simulink model "Guardian_Battery_ECM"  (R2025b)
settings: Solver=FixedStepDiscrete  StartTime=0.0  StopTime=3600  FixedStep=1  MaxStep=1  RelTol=1e-3
values from neighbouring files (symbols this model uses):
  C1 = 17000    [EKF_SOC_Estimator.m]    (also in Guardian_inputs.m)
  C2 = 5200    [Guardian_inputs.m]
  FilterDenominator = [1 -0.98]    [Guardian_inputs.m]
  FilterNumerator = [0.02]    [Guardian_inputs.m]
  NoiseLower = -0.005    [Guardian_inputs.m]
  NoiseUpper = 0.005    [Guardian_inputs.m]
  OCV_V = OCV_Table.OCV_V    [Guardian_inputs.m]
  Q_nominal = 50    [Guardian_inputs.m]
  R0 = 0.00070    (= 0.0007)    [EKF_SOC_Estimator.m]    (also in Guardian_inputs.m)
  R1 = 0.00160    (= 0.0016)    [EKF_SOC_Estimator.m]    (also in Guardian_inputs.m)
  R2 = 0.00035    [Guardian_inputs.m]
  SOC_initial = 80    [Guardian_inputs.m]
  SOC_pct = OCV_Table.SOC_pct    [Guardian_inputs.m]
  Ts = 1    [Guardian_inputs.m]
undefined symbols (not defined in the file or in its folder): dspblkCoreblockFVToolHelper, gcbh
libraries: simulink x1
settings Model: Creator=ENJAZ  LastModifiedBy=ENJAZ

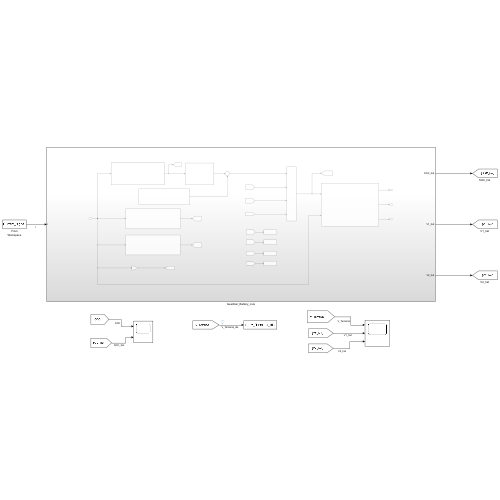
[thumbnail: Simulink's stored preview of the top-level diagram]
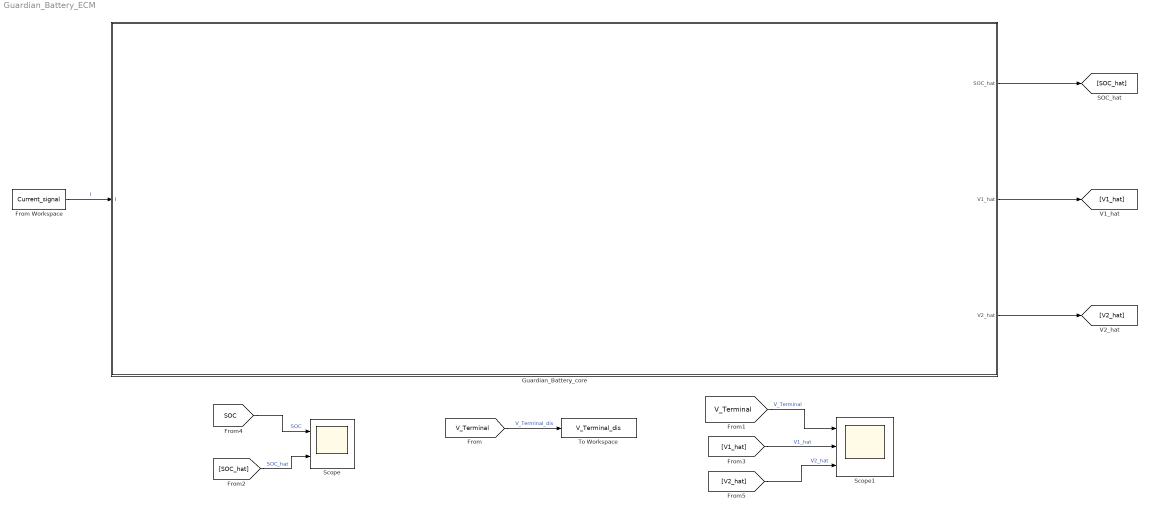
== system Guardian_Battery_ECM ==
  From Workspace : FromWorkspace  VariableName=Current_signal
  Guardian_Battery_core : Subsystem
  Scope : Scope  NumInputPorts=2
      settings: ActiveDisplayYMinimum=74.26224328559401  ActiveDisplayYMaximum=77.188865001854367
  Scope1 : Scope  NumInputPorts=3
      settings: ActiveDisplayYMinimum=-0.12940599790688978  ActiveDisplayYMaximum=0.309510284435933
  To Workspace : ToWorkspace  VariableName=V_Terminal_dis  SaveFormat=Timeseries  SampleTime=-1
  wires:
  From Workspace/1 -> Guardian_Battery_core/1(I)  "I"
  [V_Terminal] -> To Workspace/1  "V_Terminal_dis"
  [SOC] -> Scope/1  "SOC"
  [V_Terminal] -> Scope1/1  "V_Terminal"
  Guardian_Battery_core/2(V1_hat) -> [V1_hat]
  Guardian_Battery_core/1(SOC_hat) -> [SOC_hat]
  Guardian_Battery_core/3(V2_hat) -> [V2_hat]
  [SOC_hat] -> Scope/2  "SOC_hat"
  [V1_hat] -> Scope1/2  "V1_hat"
  [V2_hat] -> Scope1/3  "V2_hat"

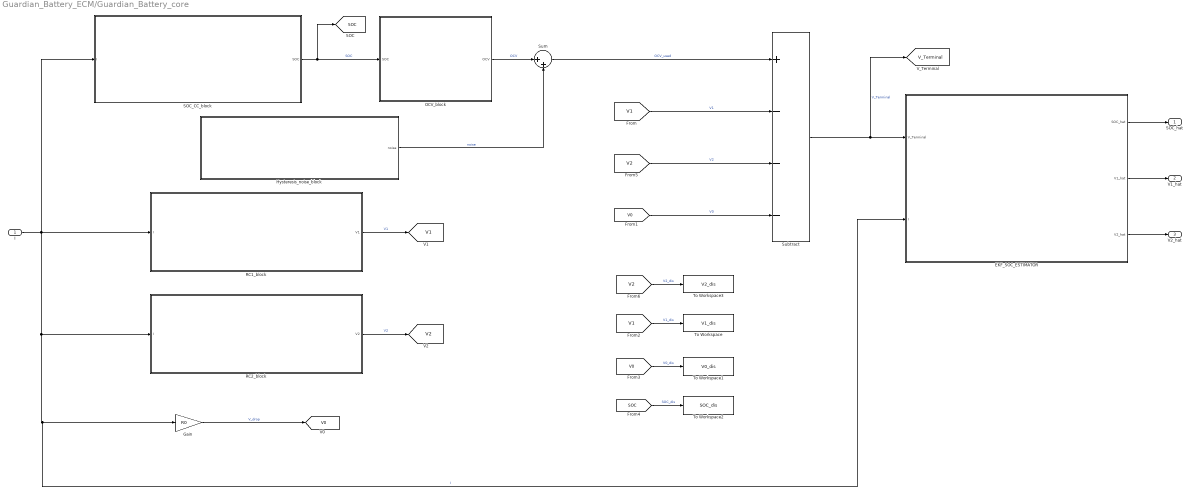
== system Guardian_Battery_ECM/Guardian_Battery_core ==
  I : Inport
  EKF_SOC_ESTIMATOR : Subsystem
  Gain : Gain  Gain=R0
  Hysteresis_noise_block : Subsystem
  OCV_block : Subsystem
  RC1_block : Subsystem
  RC2_block : Subsystem
  SOC_CC_block : Subsystem
  Subtract : Sum  Inputs=+---
  Sum : Sum  Inputs=|++
  To Workspace : ToWorkspace  VariableName=V1_dis  SaveFormat=Timeseries  SampleTime=-1
  To Workspace1 : ToWorkspace  VariableName=V0_dis  SaveFormat=Timeseries  SampleTime=-1
  To Workspace2 : ToWorkspace  VariableName=SOC_dis  SaveFormat=Timeseries  SampleTime=-1
  To Workspace3 : ToWorkspace  VariableName=V2_dis  SaveFormat=Timeseries  SampleTime=-1
  SOC_hat : Outport
  V1_hat : Outport  Port=2
  V2_hat : Outport  Port=3
  tag scope: SOC=global, V0=global, V1=global, V2=global, V_Terminal=global
  wires:
  Sum/1 -> Subtract/1  "OCV_used"
  Gain/1 -> [V0]  "V_drop"
  Subtract/1 -> EKF_SOC_ESTIMATOR/1(V_Terminal), [V_Terminal]  "V_Terminal"
  SOC_CC_block/1(SOC) -> [SOC], OCV_block/1(SOC)  "SOC"
  OCV_block/1(OCV) -> Sum/1  "OCV"
  Hysteresis_noise_block/1(noise) -> Sum/2  "noise"
  RC1_block/1(V1) -> [V1]  "V1"
  [V1] -> Subtract/2  "V1"
  [V0] -> Subtract/4  "V0"
  [V1] -> To Workspace/1  "V1_dis"
  [V0] -> To Workspace1/1  "V0_dis"
  [SOC] -> To Workspace2/1  "SOC_dis"
  RC2_block/1(V2) -> [V2]  "V2"
  I/1 -> SOC_CC_block/1(I), RC2_block/1(I), EKF_SOC_ESTIMATOR/2(I), Gain/1, RC1_block/1(I)  "I"
  [V2] -> Subtract/3  "V2"
  EKF_SOC_ESTIMATOR/1(SOC_hat) -> SOC_hat/1
  EKF_SOC_ESTIMATOR/2(V1_hat) -> V1_hat/1
  EKF_SOC_ESTIMATOR/3(V2_hat) -> V2_hat/1
  [V2] -> To Workspace3/1  "V2_dis"

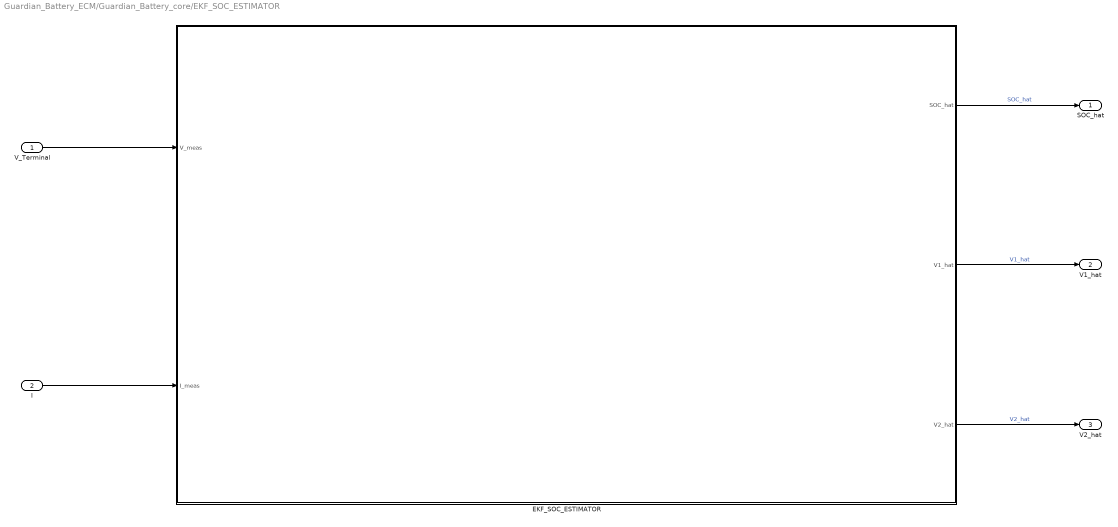
== system Guardian_Battery_ECM/Guardian_Battery_core/EKF_SOC_ESTIMATOR ==
  V_Terminal : Inport
  I : Inport  Port=2
  EKF_SOC_ESTIMATOR : MATLAB Function  TreatAsAtomicUnit=on
  SOC_hat : Outport
  V1_hat : Outport  Port=2
  V2_hat : Outport  Port=3
  wires:
  V_Terminal/1 -> EKF_SOC_ESTIMATOR/1(V_meas)
  EKF_SOC_ESTIMATOR/1(SOC_hat) -> SOC_hat/1  "SOC_hat"
  EKF_SOC_ESTIMATOR/2(V1_hat) -> V1_hat/1  "V1_hat"
  I/1 -> EKF_SOC_ESTIMATOR/2(I_meas)
  EKF_SOC_ESTIMATOR/3(V2_hat) -> V2_hat/1  "V2_hat"

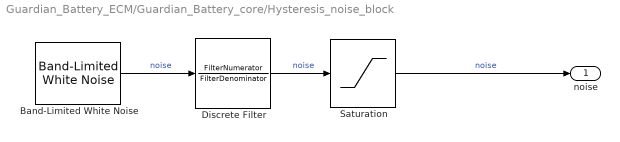
== system Guardian_Battery_ECM/Guardian_Battery_core/Hysteresis_noise_block ==
  Band-Limited White Noise : simulink/Sources/Band-Limited White Noise  Cov=[0.0001]  Ts=1  seed=[23341]
  Discrete Filter : DiscreteFilter  LoadFcn=dspblkCoreblockFVToolHelper(gcbh,'load');  Numerator=FilterNumerator  Denominator=FilterDenominator
      settings: CopyFcn=dspblkCoreblockFVToolHelper(gcbh,'copy');  DeleteFcn=dspblkCoreblockFVToolHelper(gcbh,'close');  ModelCloseFcn=dspblkCoreblockFVToolHelper(gcbh,'close');  PreSaveFcn=dspblkCoreblockFVToolHelper(gcbh,'presave');  PostSaveFcn=dspblkCoreblockFVToolHelper(gcbh,'postsave');  CloseFcn=dspblkCoreblockFVToolHelper(gcbh,'close');
  Saturation : Saturate  UpperLimit=NoiseUpper  LowerLimit=NoiseLower
  noise : Outport
  wires:
  Band-Limited White Noise/1 -> Discrete Filter/1  "noise"
  Discrete Filter/1 -> Saturation/1  "noise"
  Saturation/1 -> noise/1  "noise"

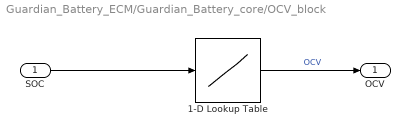
== system Guardian_Battery_ECM/Guardian_Battery_core/OCV_block ==
  SOC : Inport
  1-D Lookup Table : Lookup_n-D  NumberOfTableDimensions=1  BreakpointsForDimension1=SOC_pct  Table=OCV_V  ExtrapMethod=Clip  UseLastTableValue=on  InternalRulePriority=Speed  RndMeth=Simplest
  OCV : Outport
  wires:
  1-D Lookup Table/1 -> OCV/1  "OCV"
  SOC/1 -> 1-D Lookup Table/1

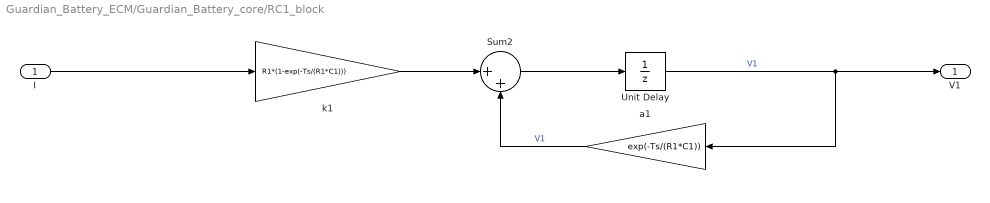
== system Guardian_Battery_ECM/Guardian_Battery_core/RC1_block ==
  I : Inport
  Sum2 : Sum  Inputs=|++
  Unit Delay : UnitDelay  SampleTime=Ts  HasFrameUpgradeWarning=on
  a1 : Gain  Gain=exp(-Ts/(R1*C1))
  k1 : Gain  Gain=R1*(1-exp(-Ts/(R1*C1)))
  V1 : Outport
  wires:
  I/1 -> k1/1
  Unit Delay/1 -> V1/1, a1/1  "V1"
  a1/1 -> Sum2/2  "V1"
  k1/1 -> Sum2/1
  Sum2/1 -> Unit Delay/1

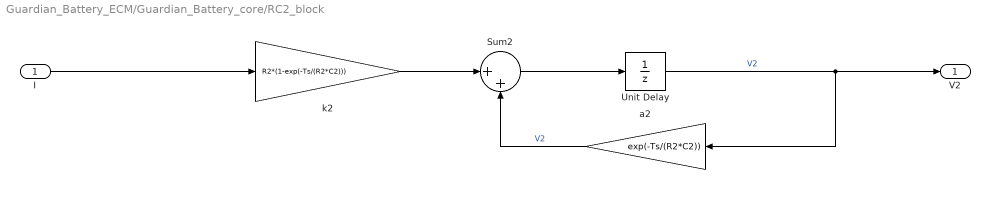
== system Guardian_Battery_ECM/Guardian_Battery_core/RC2_block ==
  I : Inport
  Sum2 : Sum  Inputs=|++
  Unit Delay : UnitDelay  SampleTime=Ts  HasFrameUpgradeWarning=on
  a2 : Gain  Gain=exp(-Ts/(R2*C2))
  k2 : Gain  Gain=R2*(1-exp(-Ts/(R2*C2)))
  V2 : Outport
  wires:
  Sum2/1 -> Unit Delay/1
  k2/1 -> Sum2/1
  a2/1 -> Sum2/2  "V2"
  Unit Delay/1 -> a2/1, V2/1  "V2"
  I/1 -> k2/1

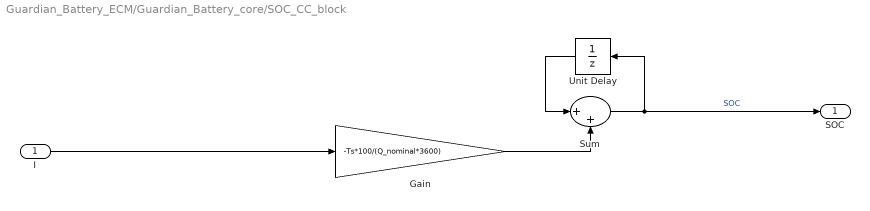
== system Guardian_Battery_ECM/Guardian_Battery_core/SOC_CC_block ==
  I : Inport
  Gain : Gain  Gain=-Ts*100/(Q_nominal*3600)
  Sum : Sum  Inputs=|++
  Unit Delay : UnitDelay  InitialCondition=SOC_initial  SampleTime=Ts  HasFrameUpgradeWarning=on
  SOC : Outport
  wires:
  Gain/1 -> Sum/2
  Sum/1 -> SOC/1, Unit Delay/1  "SOC"
  Unit Delay/1 -> Sum/1
  I/1 -> Gain/1

== matlab function Guardian_Battery_ECM/Guardian_Battery_core/EKF_SOC_ESTIMATOR/EKF_SOC_ESTIMATOR ==
  data: V_meas input; I_meas input; SOC_hat output; V1_hat output; V2_hat output
function [SOC_hat, V1_hat, V2_hat] = EKF_SOC_Estimator(V_meas, I_meas)
%EKF_SOC_ESTIMATOR  Extended Kalman Filter SOC estimator for the Guardian
%   Battery ECM Project (1RC Thevenin model, LF50K 3.2V/50Ah LFP cell).
%
%   [SOC_hat, V1_hat] = EKF_SOC_Estimator(I_meas, V_meas, Ts)
%
%   Inputs:
%     I_meas  - measured cell current (A), discharge = POSITIVE
%     V_meas  - measured terminal voltage (V)
%     Ts      - sample time (s) -- must match the model's discrete step
%
%   Outputs:
%     SOC_hat - estimated state of charge (%)
%     V1_hat  - estimated RC-branch polarization voltage (V)
%
%   THIS FILE IS PROVIDED AS-IS. Do not modify the cell parameters,
%   OCV breakpoints, or filter structure -- only the noise tuning
%   (Qcov, Rcov) and initial covariance (P0) are meant to be adjusted
%   by students, and only if they can justify the change in their report.
%
%   Usage in Simulink: paste this exact function body into a MATLAB
%   Function block with two inputs (I_meas, V_meas) and two outputs
%   (SOC_hat, V1_hat). Pass Ts as a block mask parameter or hardcode it
%   to match your model's Fixed-Step discrete sample time.
%
%   Guardian Battery ECM Project - Part 2 Addendum
%   Reference cell parameters: see project datasheet, Appendix A.

%#codegen
persistent x P initialized
if isempty(initialized)
    x = [80; 0; 0];            % initial state estimate [SOC(%); V1(V)]
                             % (80% matches the shared drive-cycle test's
                             % given initial condition -- do not change
                             % unless your report explains a cold-start
                             % scenario with an unknown initial SOC)
    P = diag([4, 0.01,0.01]);    % initial covariance
    initialized = true;
end

% ---- Fixed cell/model parameters (from project datasheet, Appendix A) ----
Q_nominal_Ah = 50;
Ts=1;
R0 = 0.00070;      % ohm  (datasheet AC impedance, 1 kHz, mid-SOC, 25 C)
R1 = 0.00160;      % ohm  (scaled from literature HPPC fit, see Appendix A)
C1 = 17000;        % F
tau1 = R1 * C1;
a = exp(-Ts / tau1);

R2 = 0.00035;      % ohm  (scaled from literature HPPC fit, see Appendix A)
C2 = 5200;        % F
tau2 = R2 * C2;
a2 = exp(-Ts / tau2);

% ---- OCV-SOC breakpoints -- MUST match Guardian_Battery_OCV_SOC_Table.csv ----
soc_bp = [0 5 10 20 30 40 50 60 70 80 90 95 100];
ocv_bp = [2.50 2.95 3.05 3.15 3.20 3.22 3.24 3.26 3.28 3.30 3.33 3.45 3.65];

% ---- Process/measurement noise tuning ----
% Qcov reflects trust in the process model (SOC integration, V1 dynamics).
% Rcov reflects trust in the voltage measurement (~20 mV sensor noise assumed).
% Students may retune these two lines; document any change and why.
Qcov = diag([1e-3, 1e-6, 1e-6]);
Rcov = 4e-4;

% =====================================================================
% PREDICT
% =====================================================================
SOC_pred = x(1) - (Ts / (Q_nominal_Ah * 3600)) * I_meas * 100;
V1_pred  = a * x(2) + R1 * (1 - a) * I_meas;
V2_pred  = a2 * x(3) + R2 * (1 - a2) * I_meas;
x_pred = [SOC_pred; V1_pred; V2_pred];

F = [1, 0,0; 0, a,0;0,0,a2];
P_pred = F * P * F' + Qcov;

% =====================================================================
% UPDATE
% =====================================================================
OCV_pred  = interp1(soc_bp, ocv_bp, x_pred(1), 'linear', 'extrap');

% Local OCV slope (finite-difference approximation of dOCV/dSOC at the
% predicted operating point) -- this is the nonlinear part of the EKF;
% a standard Kalman filter cannot handle this curved OCV(SOC) relationship.
d = 0.5;
dOCV_dSOC = interp1(soc_bp, ocv_bp, x_pred(1) + d, 'linear', 'extrap') ...
          - interp1(soc_bp, ocv_bp, x_pred(1) - d, 'linear', 'extrap');
dOCV_dSOC = dOCV_dSOC / (2 * d);

H = [dOCV_dSOC, -1,-1];

V_pred = OCV_pred - I_meas * R0 - x_pred(2)- x_pred(3);
y_resid = V_meas - V_pred;

S = H * P_pred * H' + Rcov;
K = P_pred * H' / S;

x = x_pred + K * y_resid;
P = (eye(3) - K * H) * P_pred;

% Physical bound -- SOC cannot leave [0, 100]%
x(1) = min(max(x(1), 0), 100);

SOC_hat = x(1);
V1_hat  = x(2);
V2_hat  = x(3);

end
